simulink subsystem "APPC"  (R2022b)
settings: Solver=VariableStepAuto  StartTime=0.0  StopTime=10.0  RelTol=1e-3
model mask{Max=4.5, Min=0.5}
  mask prompts: Max "Sensor Max Output Voltage (V)"; Min "Sensor Min Output Voltage (V)"
libraries: simulink x5
settings Model: DefaultTestHarness=APPS_Harness1  Creator=MAAM  LastModifiedBy=MAAM

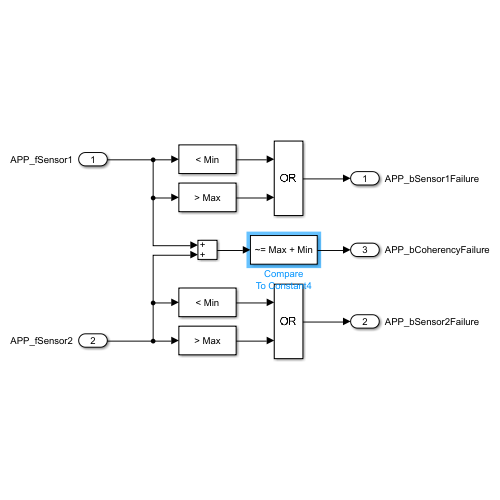
[thumbnail: Simulink's stored preview of the top-level diagram]
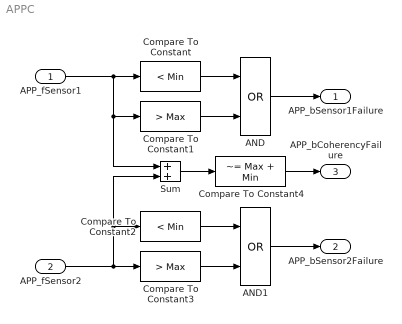
== system APPC ==
  APP_fSensor1 : Inport  OutDataTypeStr=single
  APP_fSensor2 : Inport  Port=2  OutDataTypeStr=single
  AND : Logic  Operator=OR  AllPortsSameDT=off  OutDataTypeStr=boolean
  AND1 : Logic  Operator=OR  AllPortsSameDT=off  OutDataTypeStr=boolean
  Compare To Constant : simulink/Logic and Bit Operations/Compare To Constant  relop=<  const=Min  OutDataTypeStr=boolean
  Compare To Constant1 : simulink/Logic and Bit Operations/Compare To Constant  relop=>  const=Max  OutDataTypeStr=boolean
  Compare To Constant2 : simulink/Logic and Bit Operations/Compare To Constant  relop=<  const=Min  OutDataTypeStr=boolean
  Compare To Constant3 : simulink/Logic and Bit Operations/Compare To Constant  relop=>  const=Max  OutDataTypeStr=boolean
  Compare To Constant4 : simulink/Logic and Bit Operations/Compare To Constant  relop=~=  const=Max + Min  OutDataTypeStr=boolean
  Sum : Sum
  APP_bSensor1Failure : Outport  OutDataTypeStr=boolean
  APP_bSensor2Failure : Outport  Port=2  OutDataTypeStr=boolean
  APP_bCoherencyFailure : Outport  Port=3  OutDataTypeStr=boolean
  wires:
  APP_fSensor1/1 -> Compare To Constant1/1, Sum/1, Compare To Constant/1
  Compare To Constant/1 -> AND/1
  Compare To Constant1/1 -> AND/2
  Compare To Constant3/1 -> AND1/2
  Compare To Constant2/1 -> AND1/1
  APP_fSensor2/1 -> Sum/2, Compare To Constant2/1, Compare To Constant3/1
  Sum/1 -> Compare To Constant4/1
  Compare To Constant4/1 -> APP_bCoherencyFailure/1
  AND1/1 -> APP_bSensor2Failure/1
  AND/1 -> APP_bSensor1Failure/1
